simulink model "UDPcomTest_Host"  (R2019b)
settings: Solver=FixedStepAuto  StartTime=0.0  StopTime=inf  FixedStep=0.01  RelTol=1e-3
libraries: xpcrtudplib x3, xpcutilitieslib x2, sldrtlib x1
settings Model: xpc_rtwmakecfg_data=_xpcnblib__xpcetherlib__xpcether8255xlib__xpcetherGbElib_  Creator=m.hiepp  LastModifiedBy=guy-m
settings DataIOCC: ReturnWorkspaceOutputs=off
settings DebuggingCC: ArithmeticOperatorsInVariantConditions=warning
settings SFSimCC: CustomCodeUndefinedFunction=UseInterfaceOnly

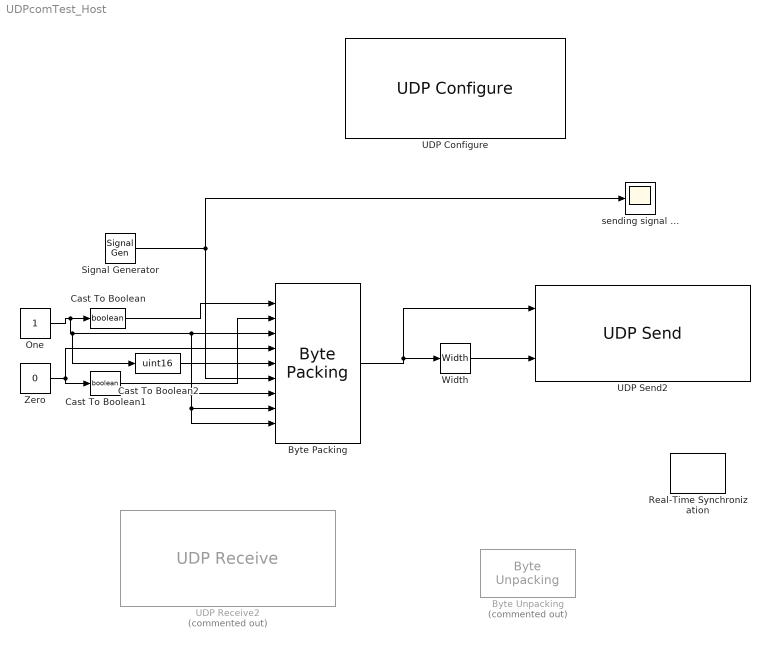
== system UDPcomTest_Host ==
  "Byte Packing " : xpcutilitieslib/Byte Packing   MaskPackedDataType=uint8  MaskUnpackedDataTypes={'boolean','boolean','double','double','uint16','double','double','double','double'}  MaskAlignment=1
  "Byte Unpacking " : xpcutilitieslib/Byte Unpacking   Commented=on  MaskUnpackedDataTypes={'uint8'}  MaskUnpackedDataSizes={[1]}  MaskAlignment=1
      settings: SourceProductName=Simulink Real-Time  SourceProductBaseCode=XP
  Cast To Boolean : DataTypeConversion  OutDataTypeStr=boolean
  Cast To Boolean1 : DataTypeConversion  OutDataTypeStr=boolean
  Cast To Boolean2 : DataTypeConversion  OutDataTypeStr=uint16
  One : Constant  OutDataTypeStr=Inherit: Inherit via back propagation
  Real-Time Synchronization : sldrtlib/Real-Time Synchronization  SampleTime=0.01  MaxMissedTicks=10  ShowMissedTicks=off  YieldWhenWaiting=off
  Signal Generator : SignalGenerator  Amplitude=10
  UDP Configure : xpcrtudplib/UDP Configure  Priority=-1  IpAddress=192.168.1.127  SubnetMask=255.255.255.0  Gateway=192.168.1.1  PciBus=0  PciSlot=0  PciFunction=0  ID=1  tune=0  disable=off  enableMulticast=off  MulticastIpAddress={}  MulticastMask={}
      settings: SourceProductName=Simulink Real-Time  SourceProductBaseCode=XP
  UDP Receive2 : xpcrtudplib/UDP Receive  Commented=on  ipAddressVal=Use host-target connection  localPort=8001  rcvWidth=16  rcvFmAny=on  fmAddress=0.0.0.0  rcvMulticast=off  multicastAddress={}  maxUDPQueue=8  sampleTime=-1
      settings: SourceProductName=Simulink Real-Time
  UDP Send2 : xpcrtudplib/UDP Send  ipAddressVal=192.168.1.127  localPort=36864  toAddress=192.168.1.156  toPort=36880  sampleTime=-1
      settings: SourceProductName=Simulink Real-Time  SourceProductBaseCode=XP
  Width : Width
  Zero : Constant  Value=0  OutDataTypeStr=Inherit: Inherit via back propagation
  sending signal ... : Scope
  wires:
  "Byte Packing "/1 -> UDP Send2/1, Width/1
  Width/1 -> UDP Send2/2
  Signal Generator/1 -> "Byte Packing "/6, sending signal .../1
  One/1 -> Cast To Boolean2/1, "Byte Packing "/9, "Byte Packing "/8, "Byte Packing "/7, "Byte Packing "/3, Cast To Boolean/1
  Zero/1 -> Cast To Boolean1/1, "Byte Packing "/4
  Cast To Boolean/1 -> "Byte Packing "/1
  Cast To Boolean1/1 -> "Byte Packing "/2
  Cast To Boolean2/1 -> "Byte Packing "/5
